simulink model "Main_Firmware_LOCAL"  (R2024b)
settings: Solver=FixedStepDiscrete  StartTime=0.0  StopTime=inf  FixedStep=sample_time  RelTol=1e-3  EnableMultiTasking=on
values from neighbouring files (symbols this model uses):
  A_f = 1.24    [Minh_Inverter_Init.m]
  C_d = 0.7041    [Minh_Inverter_Init.m]
  C_rr = 0.02    [Minh_Inverter_Init.m]
  Current_max = min(InvCurr_RMS,mCurr_RMS)*sqrt(2)    [Minh_Inverter_Init.m]
  Encoder_Offset = (PhaseA_offset/ppair)*pi/180    (= -0.785398163397)    [Minh_Inverter_Init.m]
  EPWM_F = 200000    [Minh_Inverter_Init.m]
  g = 9.8    [Minh_Inverter_Init.m]
  Inertia_z = c2d(Inertia_s, sample_time, 'zoh')    [Minh_Inverter_Init.m]
  k = 1    [Minh_Inverter_Init.m]
  lambda = 0.0375    [Minh_Inverter_Init.m]
  Ld = 0.1e-3    (= 0.0001)    [Minh_Inverter_Init.m]
  Lq = Ld    (= 0.0001)    [Minh_Inverter_Init.m]
  m = 1    [Minh_Inverter_Init.m]
  ppair = 4    [Minh_Inverter_Init.m]
  r = 0.4064/2    (= 0.2032)    [Minh_Inverter_Init.m]
  rho = 1.2    [Minh_Inverter_Init.m]
  Rs = (Rpp^2)/(Rpp*3)    (= 0.00433333333333)    [Minh_Inverter_Init.m]
  sample_time = 1/10000    (= 0.0001)    [Minh_Inverter_Init.m]
  speed_max = rpm_max*2*pi/60    (= 523.598775598)    [Minh_Inverter_Init.m]
  Torque_max = Current_max*3*lambda*ppair/2    [Minh_Inverter_Init.m]
  Voltage_max = min(V_dd,mVolt_RMS*sqrt(2))    [Minh_Inverter_Init.m]
undefined symbols (not defined in the file or in its folder): DiscIntNeverNeededParam, dspblkCoreblockFVToolHelper, gcbh, GPTRIP1SEL, TZ1
libraries: c2802xlib x8, simulink x4, slpidlib x3, spsabctodq0Lib x2, c28004xlib x1, spsdq0toabcLib x1
(part 2 of 2)

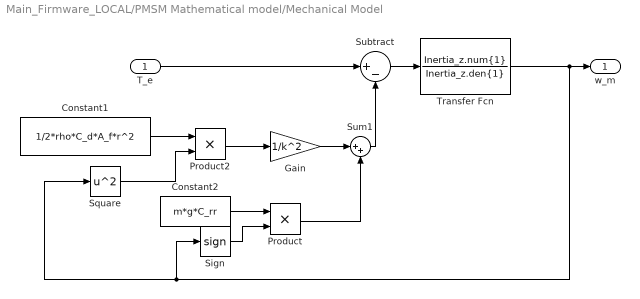
== system Main_Firmware_LOCAL/PMSM Mathematical model/Mechanical Model ==
  T_e : Inport
  Constant1 : Constant  Value=1/2*rho*C_d*A_f*r^2  OutDataTypeStr=single
  Constant2 : Constant  Value=m*g*C_rr
  Gain : Gain  Gain=1/k^2  ParamDataTypeStr=single
  Product : Product
  Product2 : Product
  Sign : Signum
  Square : Math  Operator=square  OutDataTypeStr=single
  Subtract : Sum  Inputs=|+-  OutDataTypeStr=single  RndMeth=Nearest
  Sum1 : Sum  Inputs=|++  OutDataTypeStr=single  RndMeth=Nearest
  Transfer Fcn : DiscreteTransferFcn  LoadFcn=dspblkCoreblockFVToolHelper(gcbh,'load');  Numerator=Inertia_z.num{1}  Denominator=Inertia_z.den{1}  RndMeth=Nearest  mask(DiscretizedDiscreteTransferFcn){}
      mask init:
      | %zoh
      settings: CopyFcn=dspblkCoreblockFVToolHelper(gcbh,'copy');  DeleteFcn=dspblkCoreblockFVToolHelper(gcbh,'close');  ModelCloseFcn=dspblkCoreblockFVToolHelper(gcbh,'close');  PreSaveFcn=dspblkCoreblockFVToolHelper(gcbh,'presave');  PostSaveFcn=dspblkCoreblockFVToolHelper(gcbh,'postsave');  CloseFcn=dspblkCoreblockFVToolHelper(gcbh,'close');
  w_m : Outport
  wires:
  Constant1/1 -> Product2/1
  Transfer Fcn/1 -> Sign/1, Square/1, w_m/1
  Product2/1 -> Gain/1
  Square/1 -> Product2/2
  Subtract/1 -> Transfer Fcn/1
  T_e/1 -> Subtract/1
  Sum1/1 -> Subtract/2
  Gain/1 -> Sum1/1
  Constant2/1 -> Product/1
  Sign/1 -> Product/2
  Product/1 -> Sum1/2

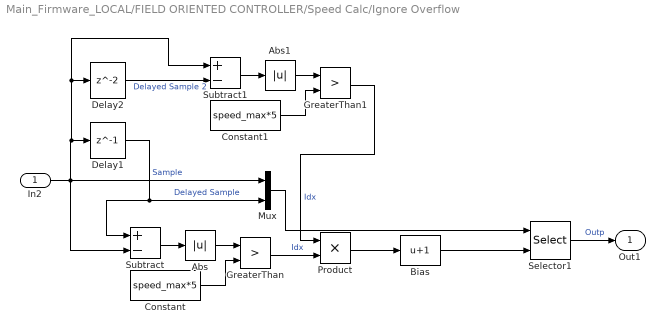
== system Main_Firmware_LOCAL/FIELD ORIENTED CONTROLLER/Speed Calc/Ignore Overflow ==
  In2 : Inport  OutDataTypeStr=single
  Abs : Abs  SaturateOnIntegerOverflow=off
  Abs1 : Abs  SaturateOnIntegerOverflow=off
  Bias : Bias  Bias=1  SaturateOnIntegerOverflow=off
  Constant : Constant  Value=speed_max*5  OutDataTypeStr=single
  Constant1 : Constant  Value=speed_max*5  OutDataTypeStr=single
  Delay1 : Delay  DelayLength=1  InputProcessing=Columns as channels (frame based)
  Delay2 : Delay  InputProcessing=Columns as channels (frame based)
  GreaterThan : RelationalOperator  Operator=>  OutDataTypeStr=fixdt(1,16)  RndMeth=Simplest  InputSameDT=off
  GreaterThan1 : RelationalOperator  Operator=>  OutDataTypeStr=fixdt(1,16)  RndMeth=Simplest  InputSameDT=off
  Mux : Mux  Inputs=2
  Product : Product
  Selector1 : Selector  InputPortWidth=2  IndexOptions=Index vector (port)  Indices=[1 3]  OutputSizes=1
  Subtract : Sum  Inputs=+-  OutDataTypeStr=single  RndMeth=Nearest
  Subtract1 : Sum  Inputs=+-  OutDataTypeStr=single  RndMeth=Nearest
  Out1 : Outport  OutDataTypeStr=single
  wires:
  In2/1 -> Subtract/2, Mux/1, Subtract1/1, Delay2/1, Delay1/1  "Sample"
  Subtract/1 -> Abs/1
  Abs/1 -> GreaterThan/1
  Constant/1 -> GreaterThan/2
  Mux/1 -> Selector1/1
  Delay1/1 -> Mux/2, Subtract/1  "Delayed Sample"
  Selector1/1 -> Out1/1  "Outp"
  Bias/1 -> Selector1/2
  Delay2/1 -> Subtract1/2  "Delayed Sample 2"
  Subtract1/1 -> Abs1/1
  Constant1/1 -> GreaterThan1/2
  Abs1/1 -> GreaterThan1/1
  GreaterThan1/1 -> Product/1  "Idx"
  Product/1 -> Bias/1
  GreaterThan/1 -> Product/2  "Idx"
